simulink model "v2_3_debug2"  (R2017a)
settings: Solver=VariableStepAuto  StartTime=0.0  StopTime=50  RelTol=1e-3
values from neighbouring files (symbols this model uses):
  EbN0 = 18    [DataForResult.mat]
libraries: commdigbbndpm3 x2, commblkintrlv2 x2, commchan3 x2, commrandsrc3 x1, dspmtrx3 x1, commsink2 x1
settings Model: Creator=DELL  LastModifiedBy=DELL

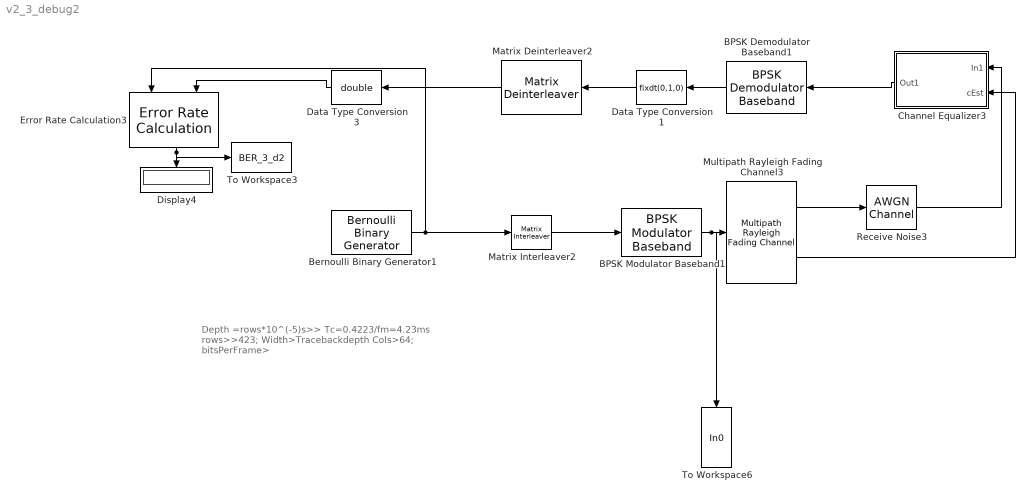
== system v2_3_debug2 ==
  note: Depth =rows*10^(-5)s>> Tc=0.4223/fm=4.23ms
      | 	rows>>423;
      |
      | Width>Tracebackdepth
      | 	Cols>64;
      |
      | bitsPerFrame>
  BPSK Demodulator Baseband1 : commdigbbndpm3/BPSK Demodulator Baseband  DecType=Hard decision  VarSource=Port  Variance=1  Ph=0  outDtype=double  derotateFactorWordLen=16  derotateFactorDataTypeStr=Inherit: Same word length as input  derotateFactorLastDataTypeStr=Inherit: Same word length as input
  BPSK Modulator Baseband1 : commdigbbndpm3/BPSK Modulator Baseband  Ph=0  outDtype=double  outWordLen=16  outUDDataType=sfix(16)  outFracLenMode=Best precision  outFracLen=15  outDataTypeStr=double  outLastDataTypeStr=double
  Bernoulli Binary Generator1 : commrandsrc3/Bernoulli Binary Generator  ProbabilityOfZero=0.5  SeedSource=Auto  Seed=0  SampleTime=1e-5  SamplesPerFrame=SamplesPerFrame  OutputDataType=double  SimulateUsing=Interpreted execution
  Channel Equalizer3 : Subsystem
      mask Display:
      | disp('Equalizer');
      | port_label('input', 2, 'cEst');
  Data Type Conversion1 : DataTypeConversion  OutDataTypeStr=fixdt(0,1,0)
  Data Type Conversion3 : DataTypeConversion  OutDataTypeStr=double
  Display4 : Display
  Error Rate Calculation3 : commsink2/Error Rate Calculation  N=0  st_delay=0  cp_mode=Entire frame  subframe=[]  PMode=Port  WsName=ErrorVec  RsMode2=off  stop=off  numErr=100  maxBits=1e6
  Matrix Deinterleaver2 : commblkintrlv2/Matrix Deinterleaver  Nrows=Rows  Ncols=Cols
      settings: SourceProductName=Communications System Toolbox  SourceProductBaseCode=CM
  Matrix Interleaver2 : commblkintrlv2/Matrix Interleaver  Nrows=Rows  Ncols=Cols
      settings: SourceProductName=Communications System Toolbox  SourceProductBaseCode=CM
  Multipath Rayleigh Fading Channel3 : commchan3/Multipath Rayleigh Fading Channel  maxDopplerShift=100  spectrumType=Jakes  sigmaGaussian=1/sqrt(2)  coeffRounded=[1 -1.72 0.785]  freqMinMaxRJakes=[0 1]  freqMinMaxAJakes=[0 1]  sigmaGaussian1=1/sqrt(2)  sigmaGaussian2=1/sqrt(2)  centerFreqGaussian1=0.0  centerFreqGaussian2=0.0  gainGaussian1=0.5  gainGaussian2=0.5  coeffBell=9  dopplerSpectrum=doppler.jakes  pathDelays=0  avgPathGaindB=2  normalizePathGains=on  seed=12345  enableProbe=0  openVisAtStart=off  outPathGains=on  outDelay=off
      settings: SourceProductName=Communications System Toolbox  SourceProductBaseCode=CM
  Receive Noise3 : commchan3/AWGN Channel  InputProcessing=Columns as channels (frame based)  seed=188  noiseMode="Signal to noise ratio  (Eb/No)"  EbNodB=EbN0  EsNodB=EbNo  SNRdB=50  bitsPerSym=1  Ps=1  Tsym=1e-5  variance=1
  To Workspace3 : ToWorkspace  VariableName=BER_3_d2  SampleTime=-1
      settings: MaxDataPoints=1
  To Workspace6 : ToWorkspace  VariableName=In0  SampleTime=-1
      settings: MaxDataPoints=1
  wires:
  BPSK Modulator Baseband1/1 -> To Workspace6/1, Multipath Rayleigh Fading Channel3/1
  Error Rate Calculation3/1 -> To Workspace3/1, Display4/1
  Multipath Rayleigh Fading Channel3/2 -> Channel Equalizer3/2(cEst)
  Multipath Rayleigh Fading Channel3/1 -> Receive Noise3/1
  Channel Equalizer3/1(Out1) -> BPSK Demodulator Baseband1/1
  Receive Noise3/1 -> Channel Equalizer3/1(In1)
  BPSK Demodulator Baseband1/1 -> Data Type Conversion1/1
  Data Type Conversion3/1 -> Error Rate Calculation3/2
  Data Type Conversion1/1 -> Matrix Deinterleaver2/1
  Bernoulli Binary Generator1/1 -> Matrix Interleaver2/1, Error Rate Calculation3/1
  Matrix Interleaver2/1 -> BPSK Modulator Baseband1/1
  Matrix Deinterleaver2/1 -> Data Type Conversion3/1

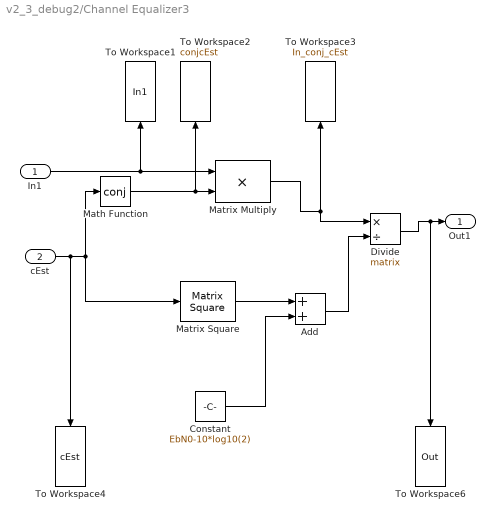
== system v2_3_debug2/Channel Equalizer3 ==
  In1 : Inport
  cEst : Inport  Port=2
  Add : Sum
  Constant : Constant  Value=EbN0-10*log10(2)
  Divide : Product  Inputs=*/  Multiplication=Matrix(*)
  Math Function : Math  Operator=conj  SaturateOnIntegerOverflow=on
  Matrix Square : dspmtrx3/Matrix Square  OutMin=[]  OutMax=[]
      settings: SourceProductName=DSP System Toolbox  SourceProductBaseCode=DS
  Matrix Multiply : Product
  To Workspace1 : ToWorkspace  VariableName=In1  SampleTime=-1
      settings: MaxDataPoints=1
  To Workspace2 : ToWorkspace  VariableName=conjcEst  SampleTime=-1
      settings: MaxDataPoints=1
  To Workspace3 : ToWorkspace  VariableName=In_conj_cEst  SampleTime=-1
      settings: MaxDataPoints=1
  To Workspace4 : ToWorkspace  VariableName=cEst  SampleTime=-1
      settings: MaxDataPoints=1
  To Workspace6 : ToWorkspace  VariableName=Out  SampleTime=-1
      settings: MaxDataPoints=1
  Out1 : Outport
  wires:
  In1/1 -> To Workspace1/1, Matrix Multiply/1
  cEst/1 -> Matrix Square/1, Math Function/1, To Workspace4/1
  Matrix Multiply/1 -> To Workspace3/1, Divide/1
  Divide/1 -> To Workspace6/1, Out1/1
  Math Function/1 -> To Workspace2/1, Matrix Multiply/2
  Matrix Square/1 -> Add/1
  Add/1 -> Divide/2
  Constant/1 -> Add/2
